simulink model "HW6_Q3_1sim"  (R2023a)
settings: Solver=VariableStepAuto  StartTime=0.0  StopTime=10  RelTol=1e-3
settings Model: Creator=USER  LastModifiedBy=USER

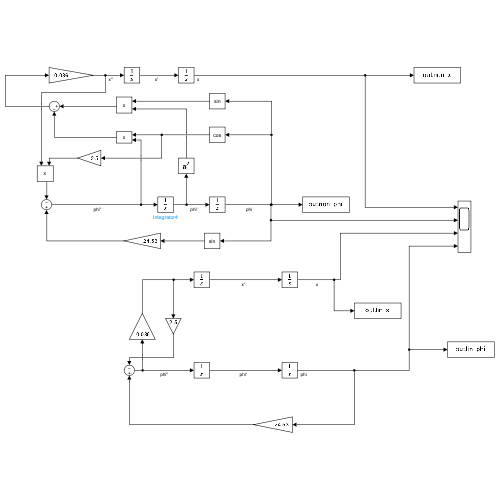
[thumbnail: Simulink's stored preview of the top-level diagram]
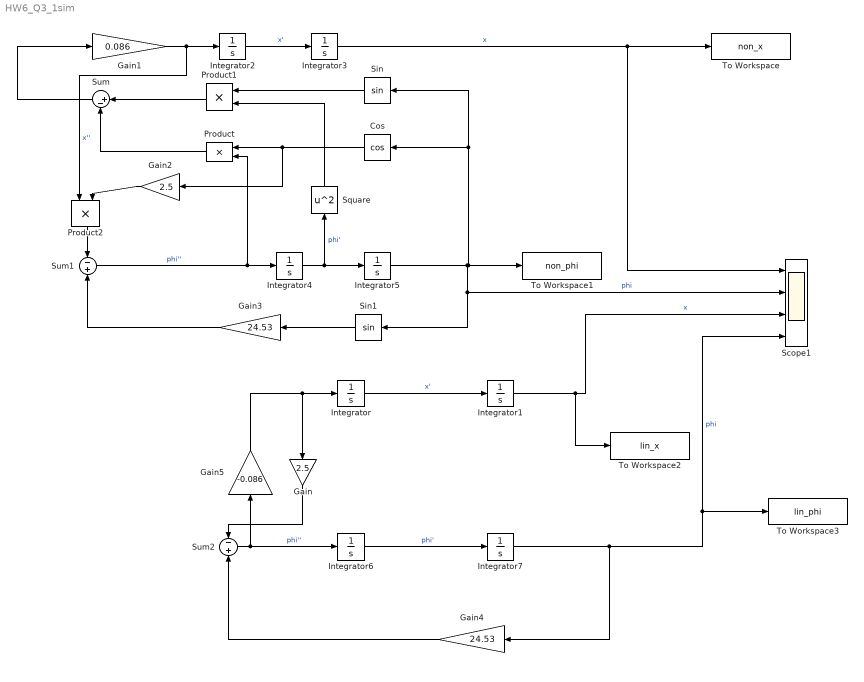
== system HW6_Q3_1sim ==
  Cos : Trigonometry  Operator=cos
  Gain : Gain  Gain=2.5
  Gain1 : Gain  Gain=0.086
  Gain2 : Gain  Gain=2.5
  Gain3 : Gain  Gain=24.53
  Gain4 : Gain  Gain=24.53
  Gain5 : Gain  Gain=-0.086
  Integrator{,1..4,6} (6 alike) : Integrator
  Integrator5 : Integrator  InitialCondition=0.1
  Integrator7 : Integrator  InitialCondition=0.1
  Product : Product
  Product1 : Product
  Product2 : Product
  Scope1 : Scope  NumInputPorts=4
  Sin : Trigonometry
  Sin1 : Trigonometry
  Square : Math  Operator=square
  Sum : Sum  Inputs=|+-
  Sum1 : Sum  Inputs=-+
  Sum2 : Sum  Inputs=-+
  To Workspace : ToWorkspace  VariableName=non_x  SaveFormat=Timeseries  SampleTime=-1
  To Workspace1 : ToWorkspace  VariableName=non_phi  SaveFormat=Timeseries  SampleTime=-1
  To Workspace2 : ToWorkspace  VariableName=lin_x  SaveFormat=Timeseries  SampleTime=-1
  To Workspace3 : ToWorkspace  VariableName=lin_phi  SaveFormat=Timeseries  SampleTime=-1
  wires:
  Integrator2/1 -> Integrator3/1  "x'"
  Integrator4/1 -> Square/1, Integrator5/1  "phi'"
  Gain1/1 -> Product2/1, Integrator2/1  "x''"
  Integrator5/1 -> To Workspace1/1, Sin/1, Cos/1, Sin1/1, Scope1/2  "phi"
  Sum1/1 -> Product/2, Integrator4/1  "phi''"
  Sum/1 -> Gain1/1
  Cos/1 -> Gain2/1, Product/1
  Product/1 -> Sum/2
  Sin/1 -> Product1/1
  Square/1 -> Product1/2
  Product1/1 -> Sum/1
  Integrator3/1 -> To Workspace/1, Scope1/1  "x"
  Product2/1 -> Sum1/1
  Gain2/1 -> Product2/2
  Sin1/1 -> Gain3/1
  Gain3/1 -> Sum1/2
  Integrator/1 -> Integrator1/1  "x'"
  Integrator1/1 -> To Workspace2/1, Scope1/3  "x"
  Integrator6/1 -> Integrator7/1  "phi'"
  Integrator7/1 -> Gain4/1, To Workspace3/1, Scope1/4  "phi"
  Sum2/1 -> Integrator6/1, Gain5/1  "phi''"
  Gain/1 -> Sum2/1
  Gain4/1 -> Sum2/2
  Gain5/1 -> Integrator/1, Gain/1
